simulink model "threeDiskOscillatorRig"  (R2023b)
settings: Solver=VariableStepAuto  StartTime=0.0  StopTime=simTime  RelTol=1e-8
values from neighbouring files (symbols this model uses):
  atan_scale = 100    [ThreeDiskOscillator.m]
  b_1 = mean(ECP_values([6 7]))    [ThreeDiskOscillator.m]    (also in rig_init.mat = 0.00287081256979)
  b_2 = mean(ECP_values([8 9]))    [ThreeDiskOscillator.m]    (also in rig_init.mat = 0.000164101446955)
  b_3 = mean(ECP_values([10 11]))    [ThreeDiskOscillator.m]    (also in rig_init.mat = 0.000179179608867)
  B_change = [1 0;0 0]    [ThreeDiskOscillator.m]
  C = [  1 0 0 0 0 0 ... (first row only)    [ThreeDiskOscillator.m]
  C_aug = [C zeros(3,1)]    [ThreeDiskOscillator.m]    (also in rig_init.mat = [1 0 0 0 0 0 0 1 0 0 0 0 ... (21 elements, 3x7)])
  C_ref = pinv(C_3*((eye(6)-F_d+G_d*K_c)^-1)*G_d*K_c)    [ThreeDiskOscillator.m]    (also in rig_init.mat = [1.24511093852 0.111747518224 0.173849858907 0.0494646296123)
  C_V_d = C_aug_v - P_V_d * C_aug_v    [ThreeDiskOscillator.m]
  den1 = cell2mat(HY3_N1_D.denominator)    [ThreeDiskOscillator.m]
  den2 = cell2mat(HY3_N2_D.denominator)    [ThreeDiskOscillator.m]
  detect_time = f_u_time + 3.75    (= 28.75)    [ThreeDiskOscillator.m]
  F_aug = [F_d G_d(:,1);zeros(1,6) 1]    [ThreeDiskOscillator.m]    (also in rig_init.mat = [0.990702941096 -4.62811422568 0.0121254081848 6.02935839899)
  f_m = [0;0;0]    [ThreeDiskOscillator.m]    (also in rig_init.mat = [0 -0.025 0])
  f_m_time = 8.5    [ThreeDiskOscillator.m]    (also in rig_init.mat)
  f_u = [0;-0.1]    [ThreeDiskOscillator.m]
  f_u_time = 25    [ThreeDiskOscillator.m]
  F_V = F_aug_v - L_V * C_aug_v    [ThreeDiskOscillator.m]
  G_aug = [G_d;0 0]    [ThreeDiskOscillator.m]    (also in rig_init.mat = [0.00334221577493 1.66717035585 6.79159923199e-06 0.00678245)
  G_V = G_aug_v    [ThreeDiskOscillator.m]
  h = double(vpasolve(eqn, h))    [ThreeDiskOscillator.m]
  J_1 = ECP_values(1)    [ThreeDiskOscillator.m]    (also in rig_init.mat = 0.00238607064451)
  J_2 = ECP_values(2)    [ThreeDiskOscillator.m]    (also in rig_init.mat = 0.00182883419357)
  J_3 = ECP_values(3)    [ThreeDiskOscillator.m]    (also in rig_init.mat = 0.00182883419357)
  k_1 = ECP_values(4)    [ThreeDiskOscillator.m]    (also in rig_init.mat = 2.78736928639)
  k_2 = ECP_values(5)    [ThreeDiskOscillator.m]    (also in rig_init.mat = 2.53389832968)
  K_c = [0.580833304421 0.052129234643 0.0810994304993 0.0230748147662 0.109041456732 0.0238388868287]    [rig_init.mat]
  L_aug = dlqe(F_aug,eye(7),C_aug,1e-3*eye(7),sigma_meas(1,1).^2*eye(3))    [ThreeDiskOscillator.m]
  num_HY1_N1_D = cell2mat(HY1_N1_D.numerator)    [ThreeDiskOscillator.m]
  num_HY2_N1_D = cell2mat(HY2_N1_D.numerator)    [ThreeDiskOscillator.m]
  num_HY2_N2_D = cell2mat(HY2_N2_D.numerator)    [ThreeDiskOscillator.m]
  num_HY3_N1_D = cell2mat(HY3_N1_D.numerator)    [ThreeDiskOscillator.m]
  num_HY3_N2_D = cell2mat(HY3_N2_D.numerator)    [ThreeDiskOscillator.m]
  P_V_d = C_aug_v * pinv(C_aug_v)    [ThreeDiskOscillator.m]
  sigma_meas = 0.0093*eye(3)    [ThreeDiskOscillator.m]    (also in rig_init.mat = [0.0093  0  0; 0  0.0093  0; 0  0  0.0093])
  T_Cm = ECP_values(13)    [ThreeDiskOscillator.m]
  T_Cp = ECP_values(12)    [ThreeDiskOscillator.m]
  T_s = 0.004    [ThreeDiskOscillator.m]    (also in rig_init.mat)
  u_fault = 1    [ThreeDiskOscillator.m]
  w_th = 0.75    [ThreeDiskOscillator.m]
  x_0 = [0;0;0;0;0;0]    [ThreeDiskOscillator.m]
undefined symbols (not defined in the file or in its folder): L_V, M
libraries: simulink x1
settings Model: Creator=dimpa  LastModifiedBy=andre
settings SolverCC: AlgebraicLoopSolver=TrustRegion
settings DataIOCC: ReturnWorkspaceOutputs=off
settings DebuggingCC: UnconnectedInputMsg=warning  UnconnectedOutputMsg=warning  UnconnectedLineMsg=warning  ArithmeticOperatorsInVariantConditions=warning
settings ModelReferenceCC: EnableRefExpFcnMdlSchedulingChecks=on
settings SFSimCC: SimUseLocalCustomCode=off  CustomCodeUndefinedFunction=UseInterfaceOnly
settings RTWCC: RTWUseLocalCustomCode=off  DLArmComputeVersion=19.05

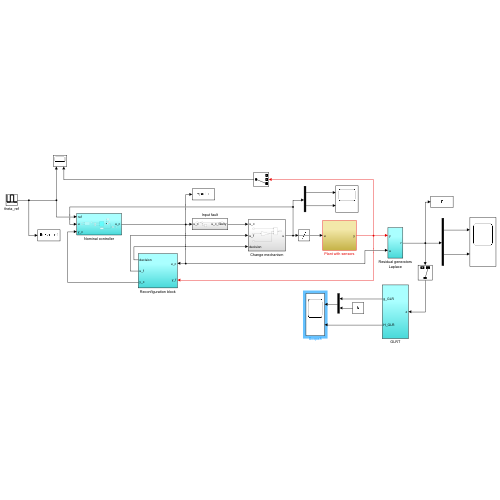
[thumbnail: Simulink's stored preview of the top-level diagram]
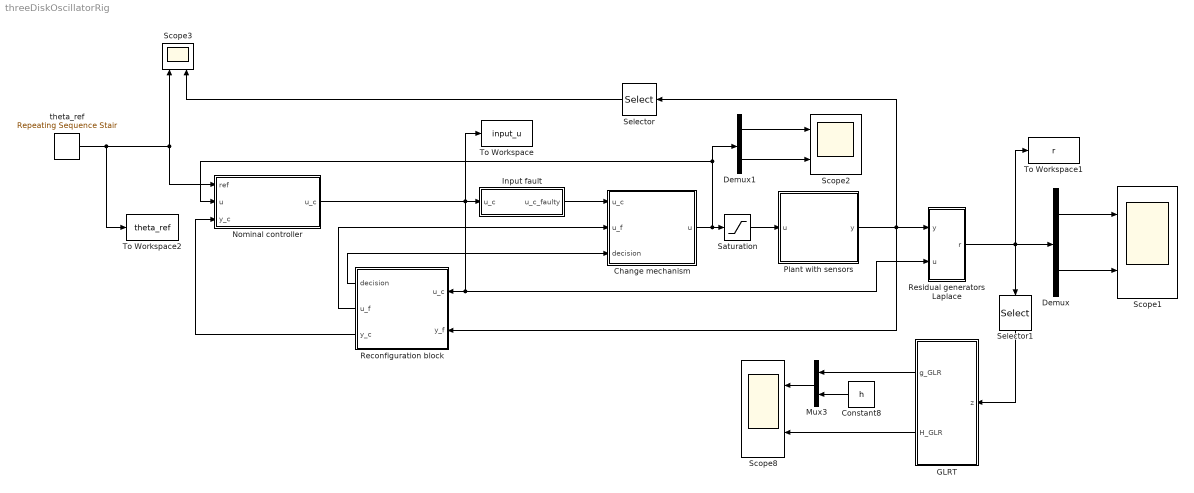
== system threeDiskOscillatorRig ==
  Change mechanism : Subsystem
  Constant8 : Constant  Value=h
  Demux : Demux  Outputs=2
  Demux1 : Demux  Outputs=2
  GLRT : Subsystem
  Input fault : Subsystem
  Mux3 : Mux  Inputs=2
  Nominal controller : Subsystem
  Plant with sensors : Subsystem
  Reconfiguration block : Subsystem
  Residual generators Laplace : Subsystem
  Saturation : Saturate  UpperLimit=2  LowerLimit=-2
  Scope{1..3,8} (4 alike) : Scope  NumInputPorts=2
  Selector : Selector  InputPortWidth=3  IndexOptions=Index vector (dialog)  Indices=[3]  OutputSizes=1
  Selector1 : Selector  InputPortWidth=2  IndexOptions=Index vector (dialog)  Indices=[2]  OutputSizes=1
  To Workspace : ToWorkspace  VariableName=input_u  SaveFormat=Timeseries  SampleTime=T_s
  To Workspace1 : ToWorkspace  VariableName=r  SaveFormat=Timeseries  SampleTime=T_s
  To Workspace2 : ToWorkspace  VariableName=theta_ref  SaveFormat=Timeseries  SampleTime=T_s
  theta_ref : simulink/Sources/Repeating Sequence Stair  OutValues=[0 1.57 0]  tsamp=5  OutMin=[]  OutMax=[]  OutDataTypeStr=double  OutputDataTypeScalingMode=double  OutDataType=fixdt(0,8)  ConRadixGroup=Best Precision: Vector-wise  OutScaling=2^-12
  wires:
  Selector/1 -> Scope3/2
  Saturation/1 -> Plant with sensors/1(u)
  theta_ref/1 -> Nominal controller/1(ref), Scope3/1, To Workspace2/1
  Plant with sensors/1(y) -> Reconfiguration block/2(y_f), Residual generators Laplace/1(y), Selector/1
  Residual generators Laplace/1(r) -> Selector1/1, Demux/1, To Workspace1/1
  GLRT/1(g_GLR) -> Mux3/1
  GLRT/2(H_GLR) -> Scope8/2
  Constant8/1 -> Mux3/2
  Mux3/1 -> Scope8/1
  Selector1/1 -> GLRT/1(z)
  Demux/1 -> Scope1/1
  Demux/2 -> Scope1/2
  Demux1/1 -> Scope2/1
  Demux1/2 -> Scope2/2
  Nominal controller/1(u_c) -> Input fault/1(u_c), Residual generators Laplace/2(u), Reconfiguration block/1(u_c), To Workspace/1
  Reconfiguration block/3(y_c) -> Nominal controller/3(y_c)
  Change mechanism/1(u) -> Nominal controller/2(u), Demux1/1, Saturation/1
  Input fault/1(u_c_faulty) -> Change mechanism/1(u_c)
  Reconfiguration block/1(decision) -> Change mechanism/3(decision)
  Reconfiguration block/2(u_f) -> Change mechanism/2(u_f)

== system threeDiskOscillatorRig/Change mechanism ==
  u_c : Inport
  u_f : Inport  Port=2
  decision : Inport  Port=3
  Gain2 : Gain  Gain=B_change  Multiplication=Matrix(K*u) (u vector)
  Switch2 : Switch  OutDataTypeStr=double  SaturateOnIntegerOverflow=off  InputSameDT=off
  u : Outport
  wires:
  Gain2/1 -> Switch2/3
  decision/1 -> Switch2/2
  u_c/1 -> Switch2/1
  Switch2/1 -> u/1
  u_f/1 -> Gain2/1

== system threeDiskOscillatorRig/GLRT ==
  z : Inport
  MATLAB Function : MATLAB Function  TreatAsAtomicUnit=on
  Unit Delay : UnitDelay  InitialCondition=zeros(M-1,1)  SampleTime=-1  HasFrameUpgradeWarning=on
  g_GLR : Outport  VectorParamsAs1DForOutWhenUnconnected=off
  H_GLR : Outport  Port=2  VectorParamsAs1DForOutWhenUnconnected=off
  wires:
  MATLAB Function/3(r_new) -> Unit Delay/1
  Unit Delay/1 -> MATLAB Function/2(r_old)
  z/1 -> MATLAB Function/1(r)
  MATLAB Function/1(g) -> g_GLR/1
  MATLAB Function/2(H) -> H_GLR/1

== system threeDiskOscillatorRig/Input fault ==
  u_c : Inport
  Sum4 : Sum  Inputs=|++
  f_u : Step  Time=f_u_time  After=f_u  SampleTime=0
  u_c_faulty : Outport
  wires:
  f_u/1 -> Sum4/2
  u_c/1 -> Sum4/1
  Sum4/1 -> u_c_faulty/1

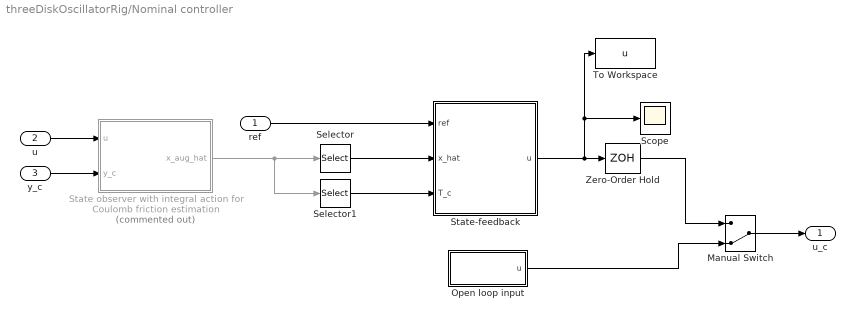
== system threeDiskOscillatorRig/Nominal controller ==
  ref : Inport
  u : Inport  Port=2
  y_c : Inport  Port=3
  Manual Switch : ManualSwitch  CurrentSetting=0
  Open loop input : Subsystem
  Scope : Scope
  Selector : Selector  InputPortWidth=7  IndexOptions=Index vector (dialog)  Indices=[1:6]  OutputSizes=1
  Selector1 : Selector  InputPortWidth=7  IndexOptions=Index vector (dialog)  Indices=[7]  OutputSizes=1
  State observer with integral action for Coulomb friction estimation : Subsystem  Commented=on
  State-feedback : Subsystem
  To Workspace : ToWorkspace  VariableName=u  SaveFormat=Timeseries  SampleTime=T_s
  Zero-Order Hold : ZeroOrderHold  SampleTime=T_s
  u_c : Outport
  wires:
  Zero-Order Hold/1 -> Manual Switch/1
  y_c/1 -> State observer with integral action for Coulomb friction estimation/2(y_c)
  u/1 -> State observer with integral action for Coulomb friction estimation/1(u)
  Open loop input/1(u) -> Manual Switch/2
  Manual Switch/1 -> u_c/1
  Selector/1 -> State-feedback/2(x_hat)
  Selector1/1 -> State-feedback/3(T_c)
  State observer with integral action for Coulomb friction estimation/1(x_aug_hat) -> Selector1/1, Selector/1
  ref/1 -> State-feedback/1(ref)
  State-feedback/1(u) -> To Workspace/1, Scope/1, Zero-Order Hold/1

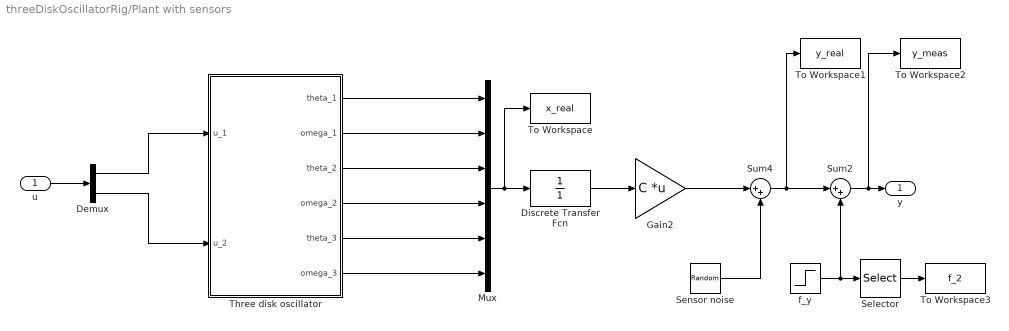
== system threeDiskOscillatorRig/Plant with sensors ==
  u : Inport
  Demux : Demux  Outputs=2
  Discrete Transfer Fcn : DiscreteTransferFcn  Denominator=[1]  SampleTime=T_s
  Gain2 : Gain  Gain=C  Multiplication=Matrix(K*u) (u vector)
  Mux : Mux  Inputs=6
  Selector : Selector  InputPortWidth=3  IndexOptions=Index vector (dialog)  Indices=[2]  OutputSizes=1
  Sensor noise : RandomNumber  Mean=zeros(3,1)  Variance=diag(sigma_meas^2)  SampleTime=T_s
  Sum2 : Sum  Inputs=|++
  Sum4 : Sum  Inputs=|++
  Three disk oscillator : Subsystem
  To Workspace : ToWorkspace  VariableName=x_real  SaveFormat=Timeseries  SampleTime=T_s
  To Workspace1 : ToWorkspace  VariableName=y_real  SaveFormat=Timeseries  SampleTime=T_s
  To Workspace2 : ToWorkspace  VariableName=y_meas  SaveFormat=Timeseries  SampleTime=T_s
  To Workspace3 : ToWorkspace  VariableName=f_2  SaveFormat=Timeseries  SampleTime=T_s
  f_y : Step  Time=f_m_time  Before=[0;0;0]  After=f_m  SampleTime=0
  y : Outport  VectorParamsAs1DForOutWhenUnconnected=off
  wires:
  u/1 -> Demux/1
  Three disk oscillator/2(omega_1) -> Mux/2
  Three disk oscillator/1(theta_1) -> Mux/1
  Mux/1 -> To Workspace/1, Discrete Transfer Fcn/1
  Three disk oscillator/4(omega_2) -> Mux/4
  Three disk oscillator/3(theta_2) -> Mux/3
  Discrete Transfer Fcn/1 -> Gain2/1
  Gain2/1 -> Sum4/1
  Sum4/1 -> To Workspace1/1, Sum2/1
  Sensor noise/1 -> Sum4/2
  Three disk oscillator/6(omega_3) -> Mux/6
  Three disk oscillator/5(theta_3) -> Mux/5
  f_y/1 -> Sum2/2, Selector/1
  Sum2/1 -> To Workspace2/1, y/1
  Selector/1 -> To Workspace3/1
  Demux/1 -> Three disk oscillator/1(u_1)
  Demux/2 -> Three disk oscillator/2(u_2)

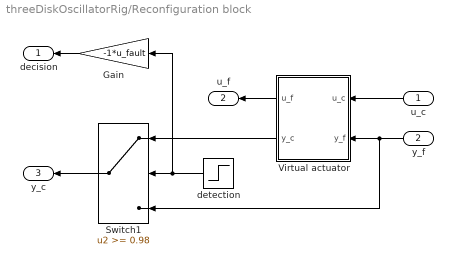
== system threeDiskOscillatorRig/Reconfiguration block ==
  u_c : Inport
  y_f : Inport  Port=2
  Gain : Gain  Gain=-1*u_fault
  Switch1 : Switch  Threshold=0.98  SaturateOnIntegerOverflow=off  InputSameDT=off
  Virtual actuator : Subsystem
  detection : Step  Time=detect_time  SampleTime=T_s
  decision : Outport  VectorParamsAs1DForOutWhenUnconnected=off
  u_f : Outport  Port=2  VectorParamsAs1DForOutWhenUnconnected=off
  y_c : Outport  Port=3  VectorParamsAs1DForOutWhenUnconnected=off
  wires:
  u_c/1 -> Virtual actuator/1(u_c)
  detection/1 -> Gain/1, Switch1/2
  Switch1/1 -> y_c/1
  Virtual actuator/2(y_c) -> Switch1/1
  y_f/1 -> Virtual actuator/2(y_f), Switch1/3
  Virtual actuator/1(u_f) -> u_f/1
  Gain/1 -> decision/1

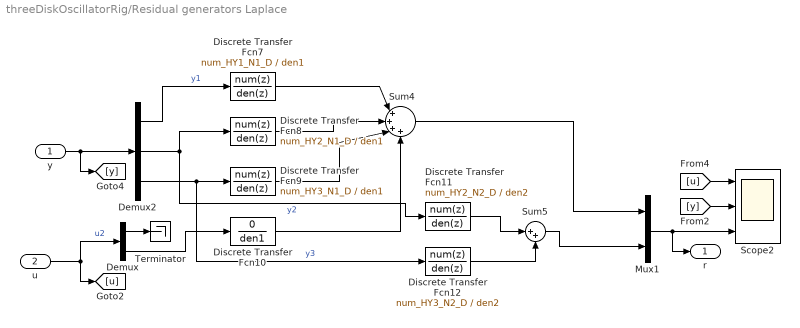
== system threeDiskOscillatorRig/Residual generators Laplace ==
  y : Inport
  u : Inport  Port=2
  Demux : Demux  Outputs=2
  Demux2 : Demux  Outputs=3
  Discrete Transfer Fcn10 : DiscreteTransferFcn  Numerator=0  Denominator=den1
  Discrete Transfer Fcn11 : DiscreteTransferFcn  Numerator=num_HY2_N2_D  Denominator=den2
  Discrete Transfer Fcn12 : DiscreteTransferFcn  Numerator=num_HY3_N2_D  Denominator=den2
  Discrete Transfer Fcn7 : DiscreteTransferFcn  Numerator=num_HY1_N1_D  Denominator=den1
  Discrete Transfer Fcn8 : DiscreteTransferFcn  Numerator=num_HY2_N1_D  Denominator=den1
  Discrete Transfer Fcn9 : DiscreteTransferFcn  Numerator=num_HY3_N1_D  Denominator=den1
  Mux1 : Mux  Inputs=2
  Scope2 : Scope  NumInputPorts=3
  Sum4 : Sum  Inputs=|++++
  Sum5 : Sum  Inputs=|++
  Terminator : Terminator
  r : Outport  VectorParamsAs1DForOutWhenUnconnected=off
  wires:
  Sum4/1 -> Mux1/1
  Mux1/1 -> Scope2/3, r/1
  y/1 -> [y], Demux2/1
  Sum5/1 -> Mux1/2
  Demux2/1 -> Discrete Transfer Fcn7/1  "y1"
  Discrete Transfer Fcn11/1 -> Sum5/1
  Discrete Transfer Fcn10/1 -> Sum4/4
  Demux2/2 -> Discrete Transfer Fcn8/1, Discrete Transfer Fcn11/1  "y2"
  Discrete Transfer Fcn12/1 -> Sum5/2
  u/1 -> [u], Demux/1  "u2"
  [u] -> Scope2/1
  [y] -> Scope2/2
  Discrete Transfer Fcn9/1 -> Sum4/3
  Demux2/3 -> Discrete Transfer Fcn12/1, Discrete Transfer Fcn9/1  "y3"
  Discrete Transfer Fcn7/1 -> Sum4/1
  Discrete Transfer Fcn8/1 -> Sum4/2
  Demux/2 -> Discrete Transfer Fcn10/1
  Demux/1 -> Terminator/1

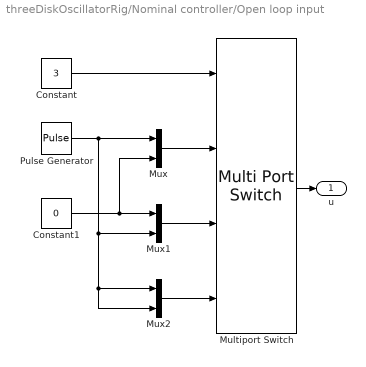
== system threeDiskOscillatorRig/Nominal controller/Open loop input ==
  Constant : Constant  Value=3
  Constant1 : Constant  Value=0
  Multiport Switch : MultiPortSwitch  SaturateOnIntegerOverflow=off  InputSameDT=off
  Mux : Mux  Inputs=2
  Mux1 : Mux  Inputs=2
  Mux2 : Mux  Inputs=2
  Pulse Generator : DiscretePulseGenerator  PulseType=Time based  Period=10  PulseWidth=5
  u : Outport
  wires:
  Constant1/1 -> Mux1/1, Mux/2
  Pulse Generator/1 -> Mux2/2, Mux2/1, Mux1/2, Mux/1
  Constant/1 -> Multiport Switch/1
  Mux2/1 -> Multiport Switch/4
  Mux/1 -> Multiport Switch/2
  Multiport Switch/1 -> u/1
  Mux1/1 -> Multiport Switch/3

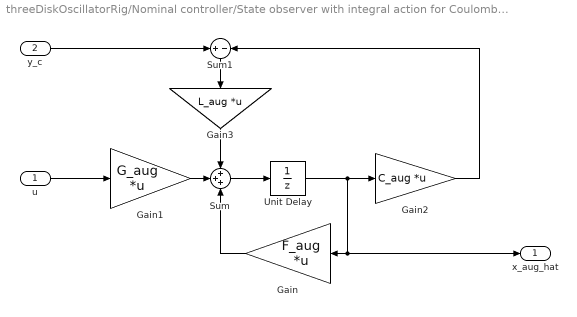
== system threeDiskOscillatorRig/Nominal controller/State observer with integral action for Coulomb friction estimation ==
  u : Inport
  y_c : Inport  Port=2
  Gain : Gain  Gain=F_aug  Multiplication=Matrix(K*u) (u vector)
  Gain1 : Gain  Gain=G_aug  Multiplication=Matrix(K*u) (u vector)
  Gain2 : Gain  Gain=C_aug  Multiplication=Matrix(K*u) (u vector)
  Gain3 : Gain  Gain=L_aug  Multiplication=Matrix(K*u) (u vector)
  Sum : Sum  Inputs=+++
  Sum1 : Sum  Inputs=+-
  Unit Delay : UnitDelay  SampleTime=T_s  HasFrameUpgradeWarning=on
  x_aug_hat : Outport  VectorParamsAs1DForOutWhenUnconnected=off
  wires:
  Unit Delay/1 -> x_aug_hat/1, Gain/1, Gain2/1
  y_c/1 -> Sum1/1
  Sum1/1 -> Gain3/1
  Sum/1 -> Unit Delay/1
  Gain2/1 -> Sum1/2
  u/1 -> Gain1/1
  Gain1/1 -> Sum/2
  Gain/1 -> Sum/3
  Gain3/1 -> Sum/1

== system threeDiskOscillatorRig/Nominal controller/State-feedback ==
  note: Feed-forward term for Coulomb friction
  ref : Inport
  x_hat : Inport  Port=2
  T_c : Inport  Port=3
  Gain2 : Gain  Gain=[1;0]
  State feedback controller : Subsystem
  Sum2 : Sum  Inputs=|+-
  u : Outport  VectorParamsAs1DForOutWhenUnconnected=off
  wires:
  T_c/1 -> Gain2/1
  Gain2/1 -> Sum2/2
  Sum2/1 -> u/1
  ref/1 -> State feedback controller/1(ref)
  x_hat/1 -> State feedback controller/2(x_hat)
  State feedback controller/1(u_fb) -> Sum2/1

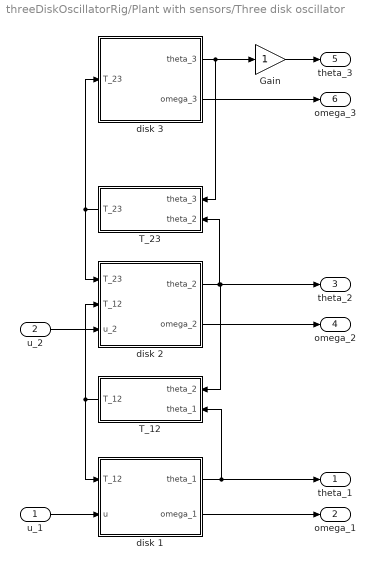
== system threeDiskOscillatorRig/Plant with sensors/Three disk oscillator ==
  u_1 : Inport
  u_2 : Inport  Port=2
  Gain : Gain
  T_12 : Subsystem
  T_23 : Subsystem
  disk 1 : Subsystem
  disk 2 : Subsystem
  disk 3 : Subsystem
  theta_1 : Outport  VectorParamsAs1DForOutWhenUnconnected=off
  omega_1 : Outport  Port=2  VectorParamsAs1DForOutWhenUnconnected=off
  theta_2 : Outport  Port=3  VectorParamsAs1DForOutWhenUnconnected=off
  omega_2 : Outport  Port=4  VectorParamsAs1DForOutWhenUnconnected=off
  theta_3 : Outport  Port=5  VectorParamsAs1DForOutWhenUnconnected=off
  omega_3 : Outport  Port=6  VectorParamsAs1DForOutWhenUnconnected=off
  wires:
  T_23/1(T_23) -> disk 2/1(T_23), disk 3/1(T_23)
  disk 1/1(theta_1) -> T_12/2(theta_1), theta_1/1
  disk 2/1(theta_2) -> T_23/2(theta_2), theta_2/1, T_12/1(theta_2)
  T_12/1(T_12) -> disk 1/1(T_12), disk 2/2(T_12)
  disk 3/2(omega_3) -> omega_3/1
  disk 1/2(omega_1) -> omega_1/1
  disk 2/2(omega_2) -> omega_2/1
  u_1/1 -> disk 1/2(u)
  disk 3/1(theta_3) -> Gain/1, T_23/1(theta_3)
  Gain/1 -> theta_3/1
  u_2/1 -> disk 2/3(u_2)

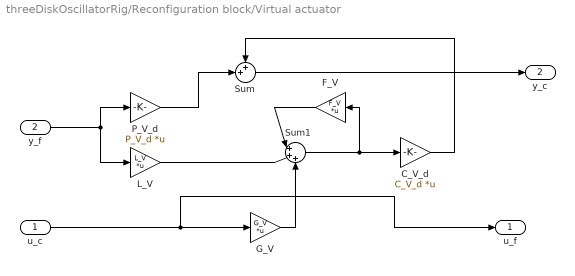
== system threeDiskOscillatorRig/Reconfiguration block/Virtual actuator ==
  u_c : Inport
  y_f : Inport  Port=2
  C_V_d : Gain  Gain=C_V_d  Multiplication=Matrix(K*u) (u vector)
  F_V : Gain  Gain=F_V  Multiplication=Matrix(K*u) (u vector)
  G_V : Gain  Gain=G_V  Multiplication=Matrix(K*u) (u vector)
  L_V : Gain  Gain=L_V  Multiplication=Matrix(K*u) (u vector)
  P_V_d : Gain  Gain=P_V_d  Multiplication=Matrix(K*u) (u vector)
  Sum : Sum  Inputs=++|
  Sum1 : Sum  Inputs=|+++
  u_f : Outport  VectorParamsAs1DForOutWhenUnconnected=off
  y_c : Outport  Port=2  VectorParamsAs1DForOutWhenUnconnected=off
  wires:
  G_V/1 -> Sum1/3
  Sum1/1 -> C_V_d/1, F_V/1
  L_V/1 -> Sum1/2
  F_V/1 -> Sum1/1
  y_f/1 -> P_V_d/1, L_V/1
  u_c/1 -> u_f/1, G_V/1
  P_V_d/1 -> Sum/2
  C_V_d/1 -> Sum/1
  Sum/1 -> y_c/1

== system threeDiskOscillatorRig/Nominal controller/State-feedback/State feedback controller ==
  ref : Inport
  x_hat : Inport  Port=2
  Gain1 : Gain  Gain=C_ref  Multiplication=Matrix(K*u) (u vector)
  Gain2 : Gain  Gain=K_c  Multiplication=Matrix(K*u) (u vector)
  Sum : Sum  Inputs=|+-
  u_fb : Outport
  wires:
  Gain1/1 -> Sum/1
  Sum/1 -> Gain2/1
  ref/1 -> Gain1/1
  x_hat/1 -> Sum/2
  Gain2/1 -> u_fb/1

== system threeDiskOscillatorRig/Plant with sensors/Three disk oscillator/T_12 ==
  theta_2 : Inport
  theta_1 : Inport  Port=2
  Gain : Gain  Gain=k_1
  Sum : Sum  Inputs=|+-
  T_12 : Outport  VectorParamsAs1DForOutWhenUnconnected=off
  wires:
  theta_2/1 -> Sum/2
  theta_1/1 -> Sum/1
  Sum/1 -> Gain/1
  Gain/1 -> T_12/1

== system threeDiskOscillatorRig/Plant with sensors/Three disk oscillator/T_23 ==
  theta_3 : Inport
  theta_2 : Inport  Port=2
  Gain : Gain  Gain=k_2
  Sum : Sum  Inputs=-+|
  T_23 : Outport  VectorParamsAs1DForOutWhenUnconnected=off
  wires:
  Gain/1 -> T_23/1
  Sum/1 -> Gain/1
  theta_3/1 -> Sum/1
  theta_2/1 -> Sum/2

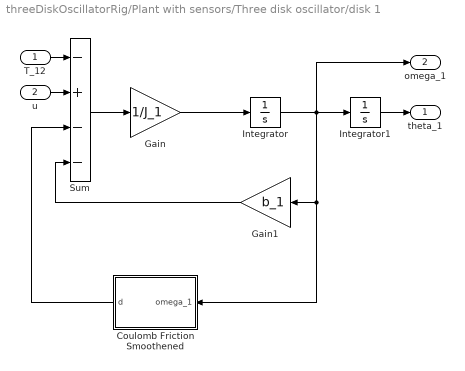
== system threeDiskOscillatorRig/Plant with sensors/Three disk oscillator/disk 1 ==
  T_12 : Inport
  u : Inport  Port=2
  Coulomb Friction Smoothened : Subsystem
  Gain : Gain  Gain=1/J_1
  Gain1 : Gain  Gain=b_1
  Integrator : Integrator  InitialCondition=x_0(2)
  Integrator1 : Integrator  InitialCondition=x_0(1)
  Sum : Sum  Inputs=-+--
  theta_1 : Outport  VectorParamsAs1DForOutWhenUnconnected=off
  omega_1 : Outport  Port=2  VectorParamsAs1DForOutWhenUnconnected=off
  wires:
  Sum/1 -> Gain/1
  Integrator/1 -> Integrator1/1, omega_1/1, Coulomb Friction Smoothened/1(omega_1), Gain1/1
  Gain1/1 -> Sum/4
  Integrator1/1 -> theta_1/1
  T_12/1 -> Sum/1
  u/1 -> Sum/2
  Gain/1 -> Integrator/1
  Coulomb Friction Smoothened/1(d) -> Sum/3

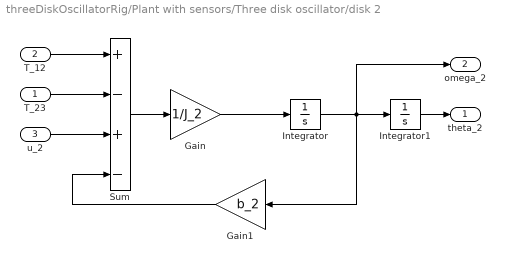
== system threeDiskOscillatorRig/Plant with sensors/Three disk oscillator/disk 2 ==
  T_23 : Inport
  T_12 : Inport  Port=2
  u_2 : Inport  Port=3
  Gain : Gain  Gain=1/J_2
  Gain1 : Gain  Gain=b_2
  Integrator : Integrator  InitialCondition=x_0(4)
  Integrator1 : Integrator  InitialCondition=x_0(3)
  Sum : Sum  Inputs=+-+-
  theta_2 : Outport  VectorParamsAs1DForOutWhenUnconnected=off
  omega_2 : Outport  Port=2  VectorParamsAs1DForOutWhenUnconnected=off
  wires:
  T_23/1 -> Sum/2
  T_12/1 -> Sum/1
  Integrator1/1 -> theta_2/1
  Gain1/1 -> Sum/4
  Gain/1 -> Integrator/1
  Integrator/1 -> Integrator1/1, Gain1/1, omega_2/1
  Sum/1 -> Gain/1
  u_2/1 -> Sum/3

== system threeDiskOscillatorRig/Plant with sensors/Three disk oscillator/disk 3 ==
  T_23 : Inport
  Gain : Gain  Gain=1/J_3
  Gain1 : Gain  Gain=b_3
  Integrator : Integrator  InitialCondition=x_0(6)
  Integrator1 : Integrator  InitialCondition=x_0(5)
  Sum : Sum  Inputs=|+-
  theta_3 : Outport  VectorParamsAs1DForOutWhenUnconnected=off
  omega_3 : Outport  Port=2  VectorParamsAs1DForOutWhenUnconnected=off
  wires:
  Sum/1 -> Gain/1
  Integrator/1 -> Integrator1/1, omega_3/1, Gain1/1
  Gain/1 -> Integrator/1
  Gain1/1 -> Sum/2
  Integrator1/1 -> theta_3/1
  T_23/1 -> Sum/1

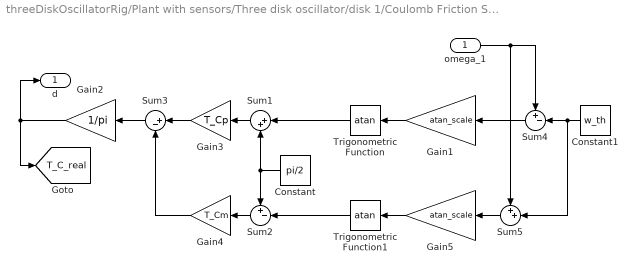
== system threeDiskOscillatorRig/Plant with sensors/Three disk oscillator/disk 1/Coulomb Friction Smoothened ==
  omega_1 : Inport
  Constant : Constant  Value=pi/2
  Constant1 : Constant  Value=w_th
  Gain1 : Gain  Gain=atan_scale
  Gain2 : Gain  Gain=1/pi
  Gain3 : Gain  Gain=T_Cp
  Gain4 : Gain  Gain=T_Cm
  Gain5 : Gain  Gain=atan_scale
  Sum1 : Sum  Inputs=|++
  Sum2 : Sum  Inputs=+-|
  Sum3 : Sum  Inputs=|+-
  Sum4 : Sum  Inputs=+-|
  Sum5 : Sum  Inputs=++|
  Trigonometric Function : Trigonometry  Operator=atan
  Trigonometric Function1 : Trigonometry  Operator=atan
  d : Outport  VectorParamsAs1DForOutWhenUnconnected=off
  tag scope: T_C_real=global
  wires:
  Gain1/1 -> Trigonometric Function/1
  Sum1/1 -> Gain3/1
  Constant/1 -> Sum2/1, Sum1/2
  Sum2/1 -> Gain4/1
  Sum3/1 -> Gain2/1
  Trigonometric Function/1 -> Sum1/1
  Gain4/1 -> Sum3/2
  Gain2/1 -> [T_C_real], d/1
  omega_1/1 -> Sum5/1, Sum4/1
  Gain3/1 -> Sum3/1
  Sum4/1 -> Gain1/1
  Constant1/1 -> Sum5/2, Sum4/2
  Gain5/1 -> Trigonometric Function1/1
  Sum5/1 -> Gain5/1
  Trigonometric Function1/1 -> Sum2/2

== matlab function threeDiskOscillatorRig/GLRT/MATLAB Function ==
  data: r input; g output size=1; H output; r_old input; r_new output
function [g, H, r_new] = GLR(r, r_old)

h = 7.568;          % h from workspace
sigma = 0.0010662;  % Sigma from workspace
M  = 10;            % M from workspace

z = [r_old(2:end); r];    % Concatenate data

maxsum = 0;
sumin=(sum(abs(z)))^2;
for j = 1:M
    sumin=(sum(abs(z)))^2;
    if sumin > maxsum
        maxsum = sumin;
    end
end
g = 1/(2 * sigma * M) * maxsum;

if g >= h
    H = 1;
else
    H = 0;
end

r_new = z(9,:);

end
